simulink model "Project26"  (R2023b)
settings: Solver=ode4  StartTime=0.0  StopTime=4*pi/n  FixedStep=0.1  RelTol=1e-3
values from neighbouring files (symbols this model uses):
  A = [A1; A2; A3; A4; A5; A6; A7; A8; A9; A10; A11; A12; A13; A14]    [Main.m]
  a = (509.4*1000+R_E+529.9*1000+R_E)/2    [Main.m]
  A_ssb = zeros(3,3,6)    [Main.m]
  e = 0.00149    [Main.m]
  epsilon = deg2rad(23.45)    [Main.m]
  F_e = 1358+600+150    (= 2108)    [Main.m]
  FOV = deg2rad(114)    [Main.m]
  G = 6.67*10^-11    (= 6.67e-11)    [Main.m]
  I = [Ix 0 0; 0 Iy 0; 0 0 Iz]    [Main.m]
  i = deg2rad(97.525)    [Main.m]
  I_inv = inv(I)    [Main.m]
  Ix = 0.13    [Main.m]
  Iy = 0.16    [Main.m]
  Iz = 0.18    [Main.m]
  j_B = [0.01, 0.05, 0.01]'    [Main.m]
  Mt = 5.97219e24    (= 5.97219e+24)    [Main.m]
  n = sqrt(G*Mt/a^3)    [Main.m]
  N_B = [n1; n2; n3; n4; n5; n6; n7; n8; n9; n10;n11;n12;n13;n14]    [Main.m]
  n_sun = 2*pi/T_earth    (= 1.99238499086e-07)    [Main.m]
  OM = deg2rad(6.934*180/12)    [Main.m]
  om = deg2rad(287.373)    [Main.m]
  q0 = [0 0 0 1]    [Main.m]
  r_CG = [0.02 0 0]    [Main.m]
  R_sun = astroConstants(2)*1e3    [Main.m]
  rF = [rF1; rF2; rF3; rF4; rF5; rF6; rF7; rF8; rF9; rF10;rF11;rF12;rF13;rF14]    [Main.m]
  theta0 = 0    [Main.m]
  Tsample = 0.1    [Main.m]
  w0 = [w_x0 w_y0 w_z0]    [Main.m]
  w_E = 7.291597763887421e-05    (= 7.29159776389e-05)    [Main.m]
  w_LN = [0 0 n]    [Main.m]
undefined symbols (not defined in the file or in its folder): actuators, control, DiscIntNeverNeededParam, environment, magnitude, sensors, settings
libraries: vrlib x6, matrix_library x5, simulink x2, aerolibutil x1
(part 2 of 2)

== system Project26/Disturbing Torques/Magnetic Torque/Rotation from Inertial to Body Frame ==
  note: $\vec{B_B} = q_{BN}'\otimes [\vec{B_N};0]\otimes q_{BN}$
  note: Quaternion Rotation (Double Tensor Product)
  q_BN : Inport
  B_N : Inport  Port=2
  Demux : Demux
  Mux : Mux  Inputs=3
  Quaternion multiplication 2 : Subsystem
  Quaternion multiplication1 : Subsystem
  To Workspace : ToWorkspace  VariableName=B_B  SampleTime=-1
  Transformation in Quaternion : Subsystem
  Transpose : Gain  Gain=[-1 -1 -1 1]
  B_B : Outport
  wires:
  B_N/1 -> Transformation in Quaternion/1(B_N)
  Mux/1 -> To Workspace/1, B_B/1
  Transpose/1 -> Quaternion multiplication1/1(q_BN)
  q_BN/1 -> Quaternion multiplication 2/2(q_BN), Transpose/1
  Transformation in Quaternion/1(q(B_N)) -> Quaternion multiplication1/2(q(B_N))
  Quaternion multiplication 2/1(q(B_B)) -> Demux/1
  Quaternion multiplication1/1(q1) -> Quaternion multiplication 2/1(q1)
  Demux/1 -> Mux/1
  Demux/2 -> Mux/2
  Demux/3 -> Mux/3

== system Project26/Kinematics/Quaternions/OMEGA Matrix ==
  note: Angular velocity
      | components
  w : Inport
  Demux : Demux  Outputs=3
  Gain1 : Gain  Gain=[0 0 0 1; 0 0 1 0; 0 -1 0 0; -1 0 0 0]
  Gain2 : Gain  Gain=[0 0 -1 0; 0 0 0 1; 1 0 0 0; 0 -1 0 0]
  Gain3 : Gain  Gain=[0 1 0 0; -1 0 0 0; 0 0 0 1; 0 0 -1 0]
  Sum : Sum  Inputs=+++
  OM Matrix : Outport
  wires:
  w/1 -> Demux/1
  Sum/1 -> OM Matrix/1
  Gain3/1 -> Sum/3
  Gain1/1 -> Sum/1
  Demux/2 -> Gain2/1
  Demux/1 -> Gain1/1
  Gain2/1 -> Sum/2
  Demux/3 -> Gain3/1

== system Project26/Orbital Mechanics and Attitude Error / Rotation from Inertial to Body Frame/Quaternion multiplication 1 ==
  q_BN' : Inport
  "q(r_N) " : Inport  Port=2
  Demux : Demux
  Gain : Gain  Gain=[1 0 0 0; 0 1 0 0; 0 0 1 0; 0 0 0 1]
  Gain1 : Gain  Gain=[0 0 0 1; 0 0 1 0 ;0 -1 0 0; -1 0 0 0]
  Gain2 : Gain  Gain=[0 0 -1 0; 0 0 0 1; 1 0 0 0; 0 -1 0 0]
  Gain3 : Gain  Gain=[0 1 0 0; -1 0 0 0; 0 0 0 1; 0 0 -1 0]
  Product : Product  Multiplication=Matrix(*)
  Sum : Sum  Inputs=|++++
  q1 : Outport
  wires:
  "q(r_N) "/1 -> Demux/1
  Demux/4 -> Gain/1
  Demux/1 -> Gain1/1
  Demux/2 -> Gain2/1
  Demux/3 -> Gain3/1
  Gain1/1 -> Sum/1
  Gain2/1 -> Sum/2
  Gain3/1 -> Sum/3
  Gain/1 -> Sum/4
  q_BN'/1 -> Product/2
  Sum/1 -> Product/1
  Product/1 -> q1/1

== system Project26/Orbital Mechanics and Attitude Error / Rotation from Inertial to Body Frame/Quaternion multiplication 2 ==
  q1 : Inport
  q_BN : Inport  Port=2
  Demux : Demux
  Gain : Gain  Gain=[1 0 0 0;0 1 0 0;0 0 1 0; 0 0 0 1]
  Gain1 : Gain  Gain=[0 0 0 1;0 0 1 0;0 -1 0 0;-1 0 0 0]
  Gain2 : Gain  Gain=[0 0 -1 0;0 0 0 1;1 0 0 0;0 -1 0 0]
  Gain3 : Gain  Gain=[0 1 0 0;-1 0 0 0;0 0 0 1;0 0 -1 0]
  Product : Product  Multiplication=Matrix(*)
  Sum : Sum  Inputs=|++++
  q(r_B) : Outport
  wires:
  q_BN/1 -> Demux/1
  Demux/4 -> Gain/1
  Demux/1 -> Gain1/1
  Demux/2 -> Gain2/1
  Demux/3 -> Gain3/1
  Gain1/1 -> Sum/1
  Gain2/1 -> Sum/2
  Gain3/1 -> Sum/3
  Gain/1 -> Sum/4
  q1/1 -> Product/2
  Sum/1 -> Product/1
  Product/1 -> q(r_B)/1

== system Project26/Orbital Mechanics and Attitude Error / Rotation from Inertial to Body Frame/Transformation in Quaternion ==
  note: Adding 0 as fourth element
      | to match the Quaternion's dimensions
  r_N : Inport
  Constant : Constant  Value=0
  Demux : Demux  Outputs=3
  Mux : Mux
  q(r_N) : Outport
  wires:
  r_N/1 -> Demux/1
  Mux/1 -> q(r_N)/1
  Constant/1 -> Mux/4
  Demux/3 -> Mux/3
  Demux/2 -> Mux/2
  Demux/1 -> Mux/1

== system Project26/Orbital Mechanics and Attitude Error /Attitude Error/Computation of q_BL ==
  note: $q_{BL} = q_{LN}'\otimes q_{BN}$
  note: Components of q_LN
  note: Tensor product to compute the error
  q_BN : Inport
  q_LN' : Inport  Port=2
  Demux : Demux
  Gain : Gain  Gain=[0,0,0,-1; 0,0,1,0; 0,-1,0,0; 1,0,0,0]
  Gain1 : Gain  Gain=[0,0,-1,0; 0,0,0,-1; 1,0,0,0; 0,1,0,0]
  Gain2 : Gain  Gain=[0, 1, 0, 0; -1, 0, 0, 0; 0, 0, 0, -1; 0, 0, 1, 0]
  Gain3 : Gain  Gain=[1,0,0,0; 0,1,0,0; 0,0,1,0; 0,0,0,1]
  Product : Product  Multiplication=Matrix(*)
  Sum : Sum  Inputs=|++++
  q_BL : Outport
  wires:
  q_LN'/1 -> Demux/1
  Demux/1 -> Gain/1
  Demux/2 -> Gain1/1
  Demux/3 -> Gain2/1
  Demux/4 -> Gain3/1
  Gain/1 -> Sum/1
  Gain1/1 -> Sum/2
  Gain2/1 -> Sum/3
  Gain3/1 -> Sum/4
  Sum/1 -> Product/1
  q_BN/1 -> Product/2
  Product/1 -> q_BL/1

== system Project26/Orbital Mechanics and Attitude Error /Attitude Error/Rotation of w_LN ==
  note: Quaternion Rotation (Double Tensor Product)
  q_BL : Inport
  w_LN : Inport  Port=2
  Demux : Demux
  Mux : Mux  Inputs=3
  Quaternion multiplication 1 : Subsystem
  Quaternion multiplication 2 : Subsystem
  To Workspace : ToWorkspace  VariableName=w_LN_B  SampleTime=-1
  Transformation in Quaternion : Subsystem
  Transpose : Gain  Gain=[-1 -1 -1 1]
  w_LN' : Outport
  wires:
  w_LN/1 -> Transformation in Quaternion/1(w_LN)
  Mux/1 -> To Workspace/1, w_LN'/1
  Transpose/1 -> Quaternion multiplication 1/1(q_BL')
  q_BL/1 -> Quaternion multiplication 2/2("q_BL "), Transpose/1
  Transformation in Quaternion/1(q_LN) -> Quaternion multiplication 1/2(q_LN)
  Quaternion multiplication 2/1(q(w_LN')) -> Demux/1
  Quaternion multiplication 1/1(q1) -> Quaternion multiplication 2/1(q1)
  Demux/1 -> Mux/1
  Demux/2 -> Mux/2
  Demux/3 -> Mux/3

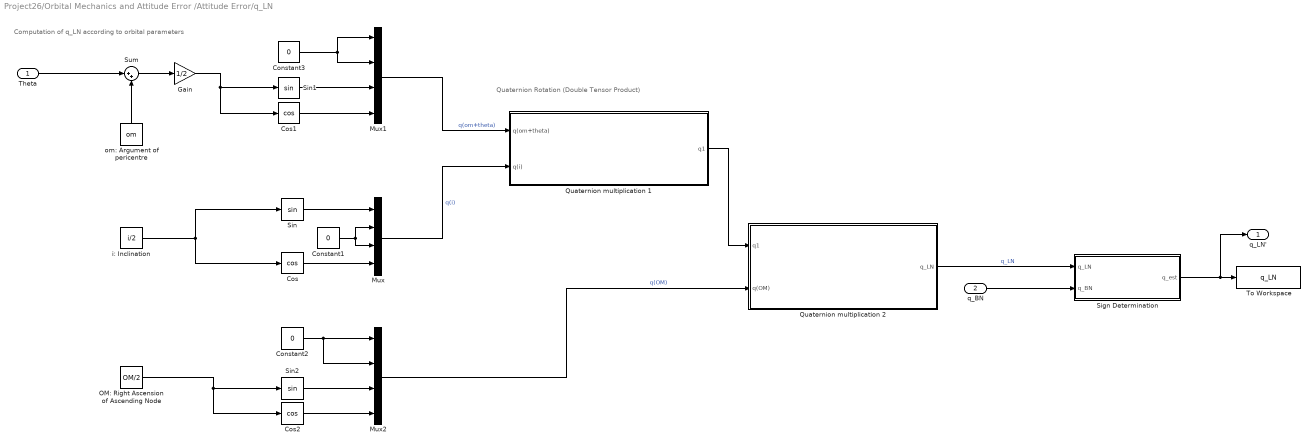
== system Project26/Orbital Mechanics and Attitude Error /Attitude Error/q_LN ==
  note: Quaternion Rotation (Double Tensor Product)
  note: Computation of q_LN according to orbital parameters
  Theta : Inport
  q_BN : Inport  Port=2
  Constant1 : Constant  Value=0
  Constant2 : Constant  Value=0
  Constant3 : Constant  Value=0
  Cos : Trigonometry  Operator=cos
  Cos1 : Trigonometry  Operator=cos
  Cos2 : Trigonometry  Operator=cos
  Gain : Gain  Gain=1/2
  Mux : Mux
  Mux1 : Mux
  Mux2 : Mux
  OM: Right Ascension of Ascending Node : Constant  Value=OM/2
  Quaternion multiplication 1 : Subsystem
  Quaternion multiplication 2 : Subsystem
  Sign Determination : Subsystem
  Sin : Trigonometry
  Sin1 : Trigonometry
  Sin2 : Trigonometry
  Sum : Sum  Inputs=|++
  To Workspace : ToWorkspace  VariableName=q_LN  SampleTime=-1
  i: Inclination : Constant  Value=i/2
  om: Argument of pericentre : Constant  Value=om
  q_LN' : Outport
  wires:
  Cos/1 -> Mux/4
  Sin/1 -> Mux/1
  Constant1/1 -> Mux/2, Mux/3
  Cos1/1 -> Mux1/4
  Constant3/1 -> Mux1/1, Mux1/2
  Sin1/1 -> Mux1/3
  Gain/1 -> Sin1/1, Cos1/1
  i: Inclination/1 -> Cos/1, Sin/1
  Theta/1 -> Sum/1
  Cos2/1 -> Mux2/4
  OM: Right Ascension of Ascending Node/1 -> Cos2/1, Sin2/1
  Sin2/1 -> Mux2/3
  Constant2/1 -> Mux2/2, Mux2/1
  om: Argument of pericentre/1 -> Sum/2
  Sum/1 -> Gain/1
  Mux1/1 -> Quaternion multiplication 1/1(q(om+theta))  "q(om+theta)"
  Mux/1 -> Quaternion multiplication 1/2(q(i))  "q(i)"
  Quaternion multiplication 1/1(q1) -> Quaternion multiplication 2/1(q1)
  Mux2/1 -> Quaternion multiplication 2/2(q(OM))  "q(OM)"
  Quaternion multiplication 2/1(q_LN) -> Sign Determination/1("q_LN ")  "q_LN"
  Sign Determination/1(q_est) -> q_LN'/1, To Workspace/1
  q_BN/1 -> Sign Determination/2(q_BN)

== system Project26/Orbital Mechanics and Attitude Error /Computation of r (vector)/Rotation (R313') from Perifocal to ECI ==
  note: $R_{313}(\Omega,i,\omega) = R_3(\omega) R_1(i)R_3(\Omega)$
  Matrix Multiply : Product  Multiplication=Matrix(*)
  Matrix Multiply1 : Product  Multiplication=Matrix(*)
  R1(i) : Constant  Value=[1 0 0;0 cos(i) sin(i) ;0 -sin(i) cos(i)]
  R3(OM) : Constant  Value=[cos(OM) sin(OM) 0; -sin(OM) cos(OM) 0; 0 0 1]
  R3(om) : Constant  Value=[cos(om) sin(om) 0;-sin(om) cos(om) 0;0 0 1]
  Transpose : Math  Operator=transpose
  Transpose1 : Math  Operator=transpose
  Transpose2 : Math  Operator=transpose
  R313 : Outport
  wires:
  R3(om)/1 -> Transpose/1
  R3(OM)/1 -> Transpose1/1
  R1(i)/1 -> Transpose2/1
  Matrix Multiply1/1 -> R313/1
  Transpose1/1 -> Matrix Multiply/1
  Transpose2/1 -> Matrix Multiply/2
  Matrix Multiply/1 -> Matrix Multiply1/1
  Transpose/1 -> Matrix Multiply1/2

== system Project26/Orbital Mechanics and Attitude Error /Rotation from Inertial to Body Frame/Quaternion multiplication 1 ==
  q_BN' : Inport
  q(S_N) : Inport  Port=2
  Demux : Demux
  Gain : Gain  Gain=[1 0 0 0; 0 1 0 0; 0 0 1 0; 0 0 0 1]
  Gain1 : Gain  Gain=[0 0 0 1; 0 0 1 0; 0 -1 0 0; -1 0 0 0]
  Gain2 : Gain  Gain=[0 0 -1 0; 0 0 0 1; 1 0 0 0; 0 -1 0 0]
  Gain3 : Gain  Gain=[0 1 0 0; -1 0 0 0; 0 0 0 1; 0 0 -1 0]
  Product : Product  Multiplication=Matrix(*)
  Sum : Sum  Inputs=|++++
  q1 : Outport
  wires:
  q(S_N)/1 -> Demux/1
  Demux/4 -> Gain/1
  Demux/1 -> Gain1/1
  Demux/2 -> Gain2/1
  Demux/3 -> Gain3/1
  Gain1/1 -> Sum/1
  Gain2/1 -> Sum/2
  Gain3/1 -> Sum/3
  Gain/1 -> Sum/4
  q_BN'/1 -> Product/2
  Sum/1 -> Product/1
  Product/1 -> q1/1

== system Project26/Orbital Mechanics and Attitude Error /Rotation from Inertial to Body Frame/Quaternion multiplication 2 ==
  q1 : Inport
  q_BN : Inport  Port=2
  Demux : Demux
  Gain : Gain  Gain=[1 0 0 0; 0 1 0 0; 0 0 1 0; 0 0 0 1]
  Gain1 : Gain  Gain=[0 0 0 1; 0 0 1 0; 0 -1 0 0; -1 0 0 0]
  Gain2 : Gain  Gain=[0 0 -1 0; 0 0 0 1; 1 0 0 0; 0 -1 0 0]
  Gain3 : Gain  Gain=[0 1 0 0; -1 0 0 0; 0 0 0 1; 0 0 -1 0]
  Product : Product  Multiplication=Matrix(*)
  Sum : Sum  Inputs=|++++
  q(S_B) : Outport
  wires:
  q_BN/1 -> Demux/1
  Demux/4 -> Gain/1
  Demux/1 -> Gain1/1
  Demux/2 -> Gain2/1
  Demux/3 -> Gain3/1
  Gain1/1 -> Sum/1
  Gain2/1 -> Sum/2
  Gain3/1 -> Sum/3
  Gain/1 -> Sum/4
  q1/1 -> Product/2
  Sum/1 -> Product/1
  Product/1 -> q(S_B)/1

== system Project26/Orbital Mechanics and Attitude Error /Rotation from Inertial to Body Frame/Transformation in Quaternion ==
  note: Adding 0 as fourth element
      | to match the Quaternion's dimensions
  S_N : Inport
  Constant : Constant  Value=0
  Demux : Demux  Outputs=3
  Mux : Mux
  q(S_N) : Outport
  wires:
  S_N/1 -> Demux/1
  Mux/1 -> q(S_N)/1
  Constant/1 -> Mux/4
  Demux/3 -> Mux/3
  Demux/2 -> Mux/2
  Demux/1 -> Mux/1

== system Project26/Sensors/Gyroscopes/Misalignment Error ==
  note: Components
  w_BN : Inport
  Cos (1) : Gain  Gain=cos(sensors.gyro.mys)
  Cos (2) : Gain  Gain=cos(sensors.gyro.mys)
  Cos (3) : Gain  Gain=cos(sensors.gyro.mys)
  Demux : Demux  Outputs=3
  Mux : Mux  Inputs=3
  Sin (1) : Gain  Gain=sin(sensors.gyro.mys/2)
  Sin (2) : Gain  Gain=sin(sensors.gyro.mys/2)
  Sin (3) : Gain  Gain=sin(sensors.gyro.mys/2)
  Sum : Sum  Inputs=|+++
  Sum1 : Sum  Inputs=|+++
  Sum2 : Sum  Inputs=|+++
  w (True Value) : Outport
  wires:
  w_BN/1 -> Demux/1
  Demux/1 -> Sin (1)/1, Cos (1)/1
  Demux/2 -> Sin (2)/1, Cos (2)/1
  Demux/3 -> Cos (3)/1, Sin (3)/1
  Cos (1)/1 -> Sum/1
  Sin (2)/1 -> Sum/2, Sum2/3
  Sin (3)/1 -> Sum/3, Sum1/3
  Cos (2)/1 -> Sum1/1
  Sin (1)/1 -> Sum2/2, Sum1/2
  Cos (3)/1 -> Sum2/1
  Sum1/1 -> Mux/2
  Sum2/1 -> Mux/3
  Sum/1 -> Mux/1
  Mux/1 -> w (True Value)/1

== system Project26/Sensors/Magnetometer/Non-Orthogonality Error ==
  note: Components
  B_B : Inport
  Cos (1) : Gain  Gain=cos(sensors.mag.mys1)
  Cos (2) : Gain  Gain=cos(sensors.mag.mys1)
  Cos (3) : Gain  Gain=cos(sensors.mag.mys1)
  Demux : Demux  Outputs=3
  Mux : Mux  Inputs=3
  Sin (1) : Gain  Gain=sin(sensors.mag.mys2)
  Sin (2) : Gain  Gain=sin(sensors.mag.mys2)
  Sin (3) : Gain  Gain=sin(sensors.mag.mys2)
  Sum : Sum  Inputs=|+++
  Sum1 : Sum  Inputs=|+++
  Sum2 : Sum  Inputs=|+++
  B_B (True) : Outport
  wires:
  B_B/1 -> Demux/1
  Demux/1 -> Cos (1)/1, Sin (1)/1
  Demux/2 -> Sin (2)/1, Cos (2)/1
  Demux/3 -> Cos (3)/1, Sin (3)/1
  Cos (1)/1 -> Sum/1
  Sin (2)/1 -> Sum2/3, Sum/2
  Sin (3)/1 -> Sum1/3, Sum/3
  Cos (2)/1 -> Sum1/1
  Sin (1)/1 -> Sum2/2, Sum1/2
  Cos (3)/1 -> Sum2/1
  Sum1/1 -> Mux/2
  Sum2/1 -> Mux/3
  Sum/1 -> Mux/1
  Mux/1 -> B_B (True)/1

== system Project26/Sensors/Sun Sensor/Angle errors ==
  alpha_x : Inport
  alpha_y : Inport  Port=2
  alpha_z : Inport  Port=3
  Constant1 : Constant  Value=[1 0 0; 0 1 0; 0 0 1]
  Gain5 : Gain  Gain=[0 0 0; 0 0 1; 0 -1 0]
  Gain6 : Gain  Gain=[0 0 -1; 0 0 0; 1 0 0]
  Gain7 : Gain  Gain=[0 1 0; -1 0 0; 0 0 0]
  Sum : Sum  Inputs=|++++
  alpha_err : Outport
  wires:
  Gain7/1 -> Sum/3
  alpha_y/1 -> Gain6/1
  Gain5/1 -> Sum/1
  alpha_x/1 -> Gain5/1
  Constant1/1 -> Sum/4
  Sum/1 -> alpha_err/1
  Gain6/1 -> Sum/2
  alpha_z/1 -> Gain7/1

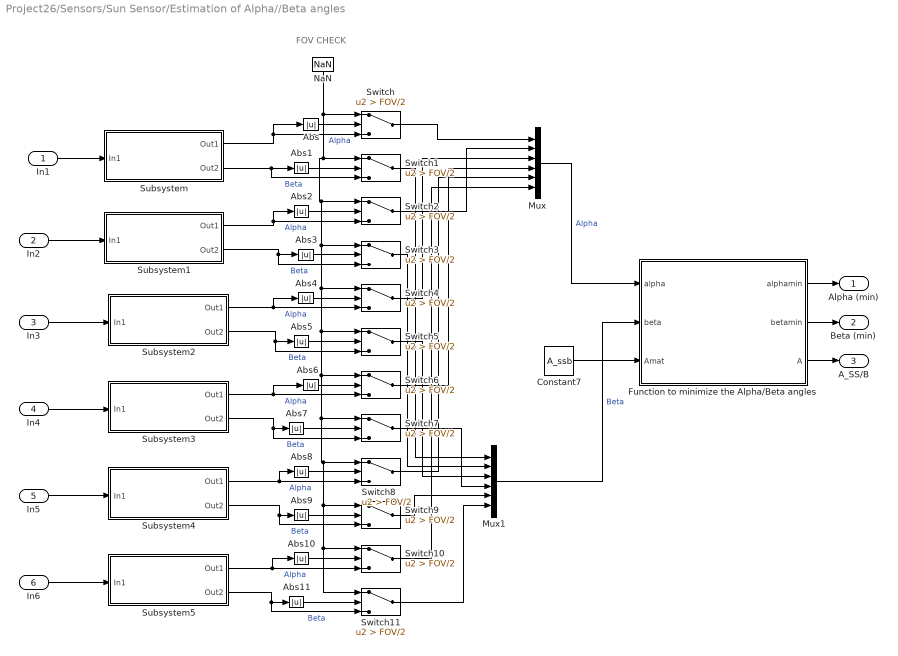
== system Project26/Sensors/Sun Sensor/Estimation of Alpha//Beta angles ==
  note: FOV CHECK
  In1 : Inport
  In2 : Inport  Port=2
  In3 : Inport  Port=3
  In4 : Inport  Port=4
  In5 : Inport  Port=5
  In6 : Inport  Port=6
  Abs{,1..11} (12 alike) : Abs  SaturateOnIntegerOverflow=off
  Constant7 : Constant  Value=A_ssb
  Function to minimize the Alpha/Beta angles : MATLAB Function  TreatAsAtomicUnit=on
  Mux : Mux  Inputs=6
  Mux1 : Mux  Inputs=6
  NaN : Constant  Value=NaN  OutDataTypeStr=Inherit: Inherit via back propagation
  Subsystem : Subsystem
  Subsystem1 : Subsystem
  Subsystem2 : Subsystem
  Subsystem3 : Subsystem
  Subsystem4 : Subsystem
  Subsystem5 : Subsystem
  Switch{,1..11} (12 alike) : Switch  Criteria=u2 > Threshold  Threshold=FOV/2  SaturateOnIntegerOverflow=off  InputSameDT=off
  Alpha (min) : Outport
  Beta (min) : Outport  Port=2
  A_SS/B : Outport  Port=3
  wires:
  Subsystem1/1(Out1) -> Abs2/1, Switch2/3  "Alpha"
  Switch6/1 -> Mux/4
  Subsystem/2(Out2) -> Switch1/3, Abs1/1  "Beta"
  In5/1 -> Subsystem4/1(In1)
  Abs10/1 -> Switch10/2
  Subsystem4/1(Out1) -> Abs8/1, Switch8/3  "Alpha"
  Abs2/1 -> Switch2/2
  Subsystem2/1(Out1) -> Abs4/1, Switch4/3  "Alpha"
  Subsystem3/1(Out1) -> Abs6/1, Switch6/3  "Alpha"
  Switch1/1 -> Mux1/1
  Abs8/1 -> Switch8/2
  Switch5/1 -> Mux1/3
  Mux/1 -> Function to minimize the Alpha/Beta angles/1(alpha)  "Alpha"
  Switch9/1 -> Mux1/5
  Subsystem2/2(Out2) -> Abs5/1, Switch5/3  "Beta"
  Abs3/1 -> Switch3/2
  Subsystem1/2(Out2) -> Abs3/1, Switch3/3  "Beta"
  Subsystem4/2(Out2) -> Switch9/3, Abs9/1  "Beta"
  Switch11/1 -> Mux1/6
  Abs6/1 -> Switch6/2
  Switch3/1 -> Mux1/2
  Abs11/1 -> Switch11/2
  Abs1/1 -> Switch1/2
  In2/1 -> Subsystem1/1(In1)
  NaN/1 -> Switch11/1, Switch10/1, Switch9/1, Switch8/1, Switch7/1, Switch6/1, Switch5/1, Switch4/1, Switch3/1, Switch2/1, Switch1/1, Switch/1
  Subsystem/1(Out1) -> Abs/1, Switch/3  "Alpha"
  Abs4/1 -> Switch4/2
  Subsystem3/2(Out2) -> Switch7/3, Abs7/1  "Beta"
  Subsystem5/1(Out1) -> Abs10/1, Switch10/3  "Alpha"
  Switch8/1 -> Mux/5
  Subsystem5/2(Out2) -> Switch11/3, Abs11/1  "Beta"
  Switch7/1 -> Mux1/4
  In6/1 -> Subsystem5/1(In1)
  Abs9/1 -> Switch9/2
  Switch2/1 -> Mux/2
  Abs7/1 -> Switch7/2
  Abs5/1 -> Switch5/2
  Switch4/1 -> Mux/3
  Switch/1 -> Mux/1
  Abs/1 -> Switch/2
  Switch10/1 -> Mux/6
  In1/1 -> Subsystem/1(In1)
  Mux1/1 -> Function to minimize the Alpha/Beta angles/2(beta)  "Beta"
  In4/1 -> Subsystem3/1(In1)
  In3/1 -> Subsystem2/1(In1)
  Function to minimize the Alpha/Beta angles/1(alphamin) -> Alpha (min)/1
  Constant7/1 -> Function to minimize the Alpha/Beta angles/3(Amat)
  Function to minimize the Alpha/Beta angles/2(betamin) -> Beta (min)/1
  Function to minimize the Alpha/Beta angles/3(A) -> A_SS/B/1

== system Project26/Attitude Determination/Enabled Subsystem/Kinematics/Quaternion ==
  note: Normalized
      | Quaternion
  w : Inport
  q_0 : Inport  Port=2
  q_BN : Inport  Port=3
  Discrete-Time Integrator : DiscreteIntegrator  InitialConditionSource=external  SampleTime=Tsample  ICPrevOutput=DiscIntNeverNeededParam  ICPrevScaledInput=DiscIntNeverNeededParam
  Gain : Gain  Gain=1/2
  Matrix Multiply : Product  Multiplication=Matrix(*)
  Omega Matrix : Subsystem
  To Workspace : ToWorkspace  VariableName=int  SampleTime=-1
  q(t) : Outport
  wires:
  Matrix Multiply/1 -> Discrete-Time Integrator/1
  Gain/1 -> Matrix Multiply/1
  w/1 -> Omega Matrix/1(In1)
  Omega Matrix/1(Out1) -> Gain/1
  q_BN/1 -> Matrix Multiply/2
  Discrete-Time Integrator/1 -> To Workspace/1, q(t)/1
  q_0/1 -> Discrete-Time Integrator/2

== system Project26/Attitude Determination/Enabled Subsystem/Kinematics/Quaternion Normalization ==
  q(t) : Inport
  Divide : Product  Inputs=*/
  Dot Product : DotProduct  OutDataTypeStr=Inherit: Inherit via internal rule
  Sqrt : Sqrt
  q_BN : Outport
  wires:
  Dot Product/1 -> Sqrt/1
  q(t)/1 -> Divide/1, Dot Product/1, Dot Product/2
  Sqrt/1 -> Divide/2
  Divide/1 -> q_BN/1

== system Project26/Attitude Determination/Enabled Subsystem/Sign Determination/Subsystem ==
  q_est : Inport
  Demux : Demux
  Mux : Mux
  Out1 : Outport
  wires:
  q_est/1 -> Demux/1
  Demux/1 -> Mux/1
  Demux/2 -> Mux/2
  Demux/3 -> Mux/3
  Demux/4 -> Mux/4
  Mux/1 -> Out1/1

== system Project26/Attitude Determination/Enabled Subsystem1/Sign determination/Subsystem ==
  q_est : Inport
  Demux : Demux
  Mux : Mux
  Out1 : Outport
  wires:
  q_est/1 -> Demux/1
  Demux/1 -> Mux/1
  Demux/2 -> Mux/2
  Demux/3 -> Mux/3
  Demux/4 -> Mux/4
  Mux/1 -> Out1/1

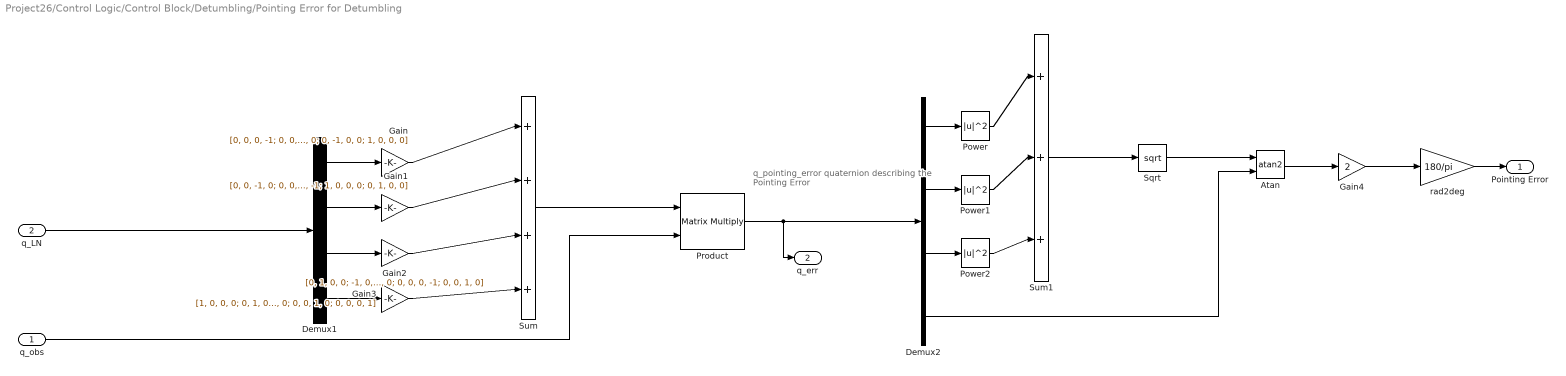
== system Project26/Control Logic/Control Block/Detumbling/Pointing Error for Detumbling ==
  note: q_pointing_error
      | quaternion describing the Pointing Error
  q_obs : Inport
  q_LN : Inport  Port=2
  Atan : Trigonometry  Operator=atan2  OutputSignalType=real
  Demux1 : Demux
  Demux2 : Demux
  Gain : Gain  Gain=[0, 0, 0, -1; 0, 0, 1, 0; 0, -1, 0, 0; 1, 0, 0, 0]
  Gain1 : Gain  Gain=[0, 0, -1, 0; 0, 0, 0, -1; 1, 0, 0, 0; 0, 1, 0, 0]
  Gain2 : Gain  Gain=[0, 1, 0, 0; -1, 0, 0, 0; 0, 0, 0, -1; 0, 0, 1, 0]
  Gain3 : Gain  Gain=[1, 0, 0, 0; 0, 1, 0, 0; 0, 0, 1, 0; 0, 0, 0, 1]
  Gain4 : Gain  Gain=2
  Power : Math  Operator=magnitude^2
  Power1 : Math  Operator=magnitude^2
  Power2 : Math  Operator=magnitude^2
  Product : Product  Multiplication=Matrix(*)
  Sqrt : Sqrt
  Sum : Sum  Inputs=|++++
  Sum1 : Sum  Inputs=|+++
  rad2deg : Gain  Gain=180/pi
  Pointing Error : Outport
  q_err : Outport  Port=2
  wires:
  Power1/1 -> Sum1/2
  Demux2/4 -> Atan/2
  Atan/1 -> Gain4/1
  Power/1 -> Sum1/1
  Demux2/2 -> Power1/1
  Demux2/3 -> Power2/1
  Demux2/1 -> Power/1
  Sum1/1 -> Sqrt/1
  Power2/1 -> Sum1/3
  Sqrt/1 -> Atan/1
  Product/1 -> q_err/1, Demux2/1
  Gain/1 -> Sum/1
  Gain2/1 -> Sum/3
  Gain1/1 -> Sum/2
  Demux1/3 -> Gain2/1
  Demux1/1 -> Gain/1
  Gain3/1 -> Sum/4
  Demux1/2 -> Gain1/1
  Demux1/4 -> Gain3/1
  Sum/1 -> Product/1
  rad2deg/1 -> Pointing Error/1
  q_LN/1 -> Demux1/1
  Gain4/1 -> rad2deg/1
  q_obs/1 -> Product/2

== system Project26/Control Logic/Control Block/Detumbling/Rotation of w_DET ==
  note: Quaternion Rotation (Double Tensor Product)
  w_DET : Inport
  q_err : Inport  Port=2
  Demux : Demux
  Mux : Mux  Inputs=3
  Quaternion multiplication 1 : Subsystem
  Quaternion multiplication 2 : Subsystem
  Transformation in Quaternion : Subsystem
  Transpose : Gain  Gain=[-1 -1 -1 1]
  w_det_body : Outport
  wires:
  w_DET/1 -> Transformation in Quaternion/1(w_LN)
  Mux/1 -> w_det_body/1
  Transpose/1 -> Quaternion multiplication 1/1(q_BL' = q)
  q_err/1 -> Quaternion multiplication 2/2(q_BL = q'), Transpose/1
  Transformation in Quaternion/1(q_LN) -> Quaternion multiplication 1/2(q_LN = q')
  Quaternion multiplication 2/1(q*q' = q2) -> Demux/1
  Quaternion multiplication 1/1(q*q' = q1) -> Quaternion multiplication 2/1(q1 = q)
  Demux/1 -> Mux/1
  Demux/2 -> Mux/2
  Demux/3 -> Mux/3

== system Project26/Control Logic/Control Block/Slew Maneuvre/Pointing Error for Slew Maneuvre ==
  note: q_pointing_error
      | quaternion describing the Pointing Error
  q_LN : Inport
  q_obs : Inport  Port=2
  Atan : Trigonometry  Operator=atan2  OutputSignalType=real
  Demux1 : Demux
  Demux2 : Demux
  Gain : Gain  Gain=[0, 0, 0, -1; 0, 0, 1, 0; 0, -1, 0, 0; 1, 0, 0, 0]
  Gain1 : Gain  Gain=[0, 0, -1, 0; 0, 0, 0, -1; 1, 0, 0, 0; 0, 1, 0, 0]
  Gain2 : Gain  Gain=[0, 1, 0, 0; -1, 0, 0, 0; 0, 0, 0, -1; 0, 0, 1, 0]
  Gain3 : Gain  Gain=[1, 0, 0, 0; 0, 1, 0, 0; 0, 0, 1, 0; 0, 0, 0, 1]
  Gain4 : Gain  Gain=2
  Power : Math  Operator=magnitude^2
  Power1 : Math  Operator=magnitude^2
  Power2 : Math  Operator=magnitude^2
  Product : Product  Multiplication=Matrix(*)
  Sqrt : Sqrt
  Sum : Sum  Inputs=|++++
  Sum1 : Sum  Inputs=|+++
  rad2deg : Gain  Gain=180/pi
  Pointing Error : Outport
  q_e : Outport  Port=2
  wires:
  Power1/1 -> Sum1/2
  Demux2/4 -> Atan/2
  Atan/1 -> rad2deg/1
  Power/1 -> Sum1/1
  Demux2/2 -> Power1/1
  Demux2/3 -> Power2/1
  Demux2/1 -> Power/1
  Sum1/1 -> Sqrt/1
  Power2/1 -> Sum1/3
  Sqrt/1 -> Atan/1
  Product/1 -> Demux2/1, q_e/1
  Gain/1 -> Sum/1
  Gain2/1 -> Sum/3
  Gain1/1 -> Sum/2
  Demux1/3 -> Gain2/1
  Demux1/1 -> Gain/1
  Gain3/1 -> Sum/4
  Demux1/2 -> Gain1/1
  Demux1/4 -> Gain3/1
  Sum/1 -> Product/1
  rad2deg/1 -> Gain4/1
  q_LN/1 -> Demux1/1
  Gain4/1 -> Pointing Error/1
  q_obs/1 -> Product/2

== system Project26/Control Logic/Control Block/Slew Maneuvre/Rotation of w_SM ==
  note: Quaternion Rotation (Double Tensor Product)
  w_SM : Inport
  q_e : Inport  Port=2
  Demux : Demux
  Mux : Mux  Inputs=3
  Quaternion multiplication 1 : Subsystem
  Quaternion multiplication 2 : Subsystem
  Transformation in Quaternion : Subsystem
  Transpose : Gain  Gain=[-1 -1 -1 1]
  w_SM_body : Outport
  wires:
  w_SM/1 -> Transformation in Quaternion/1(w_LN)
  Mux/1 -> w_SM_body/1
  Transpose/1 -> Quaternion multiplication 1/1(q_BL')
  q_e/1 -> Quaternion multiplication 2/2(q_BL), Transpose/1
  Transformation in Quaternion/1(q_LN) -> Quaternion multiplication 1/2(q_LN)
  Quaternion multiplication 2/1(q(w_SM_B)) -> Demux/1
  Quaternion multiplication 1/1(q1) -> Quaternion multiplication 2/1(q1)
  Demux/1 -> Mux/1
  Demux/2 -> Mux/2
  Demux/3 -> Mux/3

== system Project26/Control Logic/Control Block/Trajectory Tracking/Conversion from quaternions to DCM ==
  note: q*q^t
  note: Matrix I
  note: q^tq
  note: q^t
  q_err : Inport
  Demux : Demux
  Gain : Gain  Gain=-2
  Gain1 : Gain  Gain=[1 0 0;0 1 0;0 0 1]
  Gain2 : Gain  Gain=2
  Matrix Multiply : Product  Multiplication=Matrix(*)
  Mux : Mux  Inputs=3
  Product : Product  Multiplication=Matrix(*)
  Product1 : Product
  Square : Math  Operator=square
  Sum : Sum  Inputs=|-+
  Sum1 : Sum  Inputs=|+++
  Transpose : Math  Operator=transpose
  "[q^] matrix" : Subsystem
  A_e : Outport
  wires:
  q_err/1 -> Demux/1
  Demux/1 -> Mux/1, "[q^] matrix"/1(In1)
  Demux/2 -> Mux/2, "[q^] matrix"/2(In2)
  Demux/4 -> Square/1, Gain/1
  Demux/3 -> Mux/3, "[q^] matrix"/3(In3)
  Square/1 -> Sum/2
  Sum/1 -> Gain1/1
  Gain2/1 -> Sum1/1
  Product1/1 -> Sum1/2
  Gain1/1 -> Sum1/3
  Sum1/1 -> A_e/1
  "[q^] matrix"/1(Out1) -> Product1/2
  Gain/1 -> Product1/1
  Transpose/1 -> Product/1, Matrix Multiply/2
  Product/1 -> Sum/1
  Mux/1 -> Matrix Multiply/1, Product/2, Transpose/1
  Matrix Multiply/1 -> Gain2/1

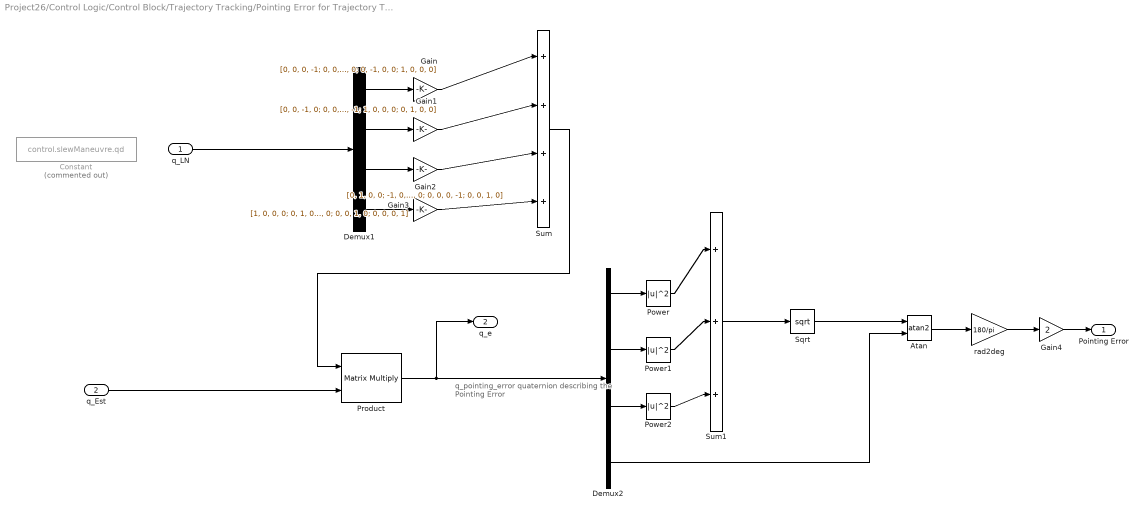
== system Project26/Control Logic/Control Block/Trajectory Tracking/Pointing Error for Trajectory Tracking ==
  note: q_pointing_error
      | quaternion describing the Pointing Error
  q_LN : Inport
  q_Est : Inport  Port=2
  Atan : Trigonometry  Operator=atan2  OutputSignalType=real
  Constant : Constant  Commented=on  Value=control.slewManeuvre.qd
  Demux1 : Demux
  Demux2 : Demux
  Gain : Gain  Gain=[0, 0, 0, -1; 0, 0, 1, 0; 0, -1, 0, 0; 1, 0, 0, 0]
  Gain1 : Gain  Gain=[0, 0, -1, 0; 0, 0, 0, -1; 1, 0, 0, 0; 0, 1, 0, 0]
  Gain2 : Gain  Gain=[0, 1, 0, 0; -1, 0, 0, 0; 0, 0, 0, -1; 0, 0, 1, 0]
  Gain3 : Gain  Gain=[1, 0, 0, 0; 0, 1, 0, 0; 0, 0, 1, 0; 0, 0, 0, 1]
  Gain4 : Gain  Gain=2
  Power : Math  Operator=magnitude^2
  Power1 : Math  Operator=magnitude^2
  Power2 : Math  Operator=magnitude^2
  Product : Product  Multiplication=Matrix(*)
  Sqrt : Sqrt
  Sum : Sum  Inputs=|++++
  Sum1 : Sum  Inputs=|+++
  rad2deg : Gain  Gain=180/pi
  Pointing Error : Outport
  q_e : Outport  Port=2
  wires:
  Power1/1 -> Sum1/2
  Demux2/4 -> Atan/2
  Atan/1 -> rad2deg/1
  Power/1 -> Sum1/1
  Demux2/2 -> Power1/1
  Demux2/3 -> Power2/1
  Demux2/1 -> Power/1
  Sum1/1 -> Sqrt/1
  Power2/1 -> Sum1/3
  Sqrt/1 -> Atan/1
  Product/1 -> Demux2/1, q_e/1
  Gain/1 -> Sum/1
  Gain2/1 -> Sum/3
  Gain1/1 -> Sum/2
  Demux1/3 -> Gain2/1
  Demux1/1 -> Gain/1
  Gain3/1 -> Sum/4
  Demux1/2 -> Gain1/1
  Demux1/4 -> Gain3/1
  Sum/1 -> Product/1
  rad2deg/1 -> Gain4/1
  q_LN/1 -> Demux1/1
  Gain4/1 -> Pointing Error/1
  q_Est/1 -> Product/2

== system Project26/Disturbing Torques/Gravity Gradient Torque/Rotation of vector [1 0 0]/Quaternion multiplication 1 ==
  q_BL : Inport
  q(vect) : Inport  Port=2
  Demux : Demux
  Gain : Gain  Gain=[1 0 0 0; 0 1 0 0; 0 0 1 0; 0 0 0 1]
  Gain1 : Gain  Gain=[0 0 0 1; 0 0 1 0; 0 -1 0 0; -1 0 0 0]
  Gain2 : Gain  Gain=[0 0 -1 0; 0 0 0 1; 1 0 0 0; 0 -1 0 0]
  Gain3 : Gain  Gain=[0 1 0 0; -1 0 0 0; 0 0 0 1; 0 0 -1 0]
  Product : Product  Multiplication=Matrix(*)
  Sum : Sum  Inputs=|++++
  q1 : Outport
  wires:
  q(vect)/1 -> Demux/1
  Demux/4 -> Gain/1
  Demux/1 -> Gain1/1
  Demux/2 -> Gain2/1
  Demux/3 -> Gain3/1
  Gain1/1 -> Sum/1
  Gain2/1 -> Sum/2
  Gain3/1 -> Sum/3
  Gain/1 -> Sum/4
  q_BL/1 -> Product/2
  Sum/1 -> Product/1
  Product/1 -> q1/1

== system Project26/Disturbing Torques/Gravity Gradient Torque/Rotation of vector [1 0 0]/Quaternion multiplication 2 ==
  q1 : Inport
  q_BL : Inport  Port=2
  Demux : Demux
  Gain : Gain  Gain=[1 0 0 0; 0 1 0 0; 0 0 1 0; 0 0 0 1]
  Gain1 : Gain  Gain=[0 0 0 1; 0 0 1 0; 0 -1 0 0; -1 0 0 0]
  Gain2 : Gain  Gain=[0 0 -1 0; 0 0 0 1; 1 0 0 0; 0 -1 0 0]
  Gain3 : Gain  Gain=[0 1 0 0; -1 0 0 0; 0 0 0 1; 0 0 -1 0]
  Product : Product  Multiplication=Matrix(*)
  Sum : Sum  Inputs=|++++
  q(v_rot) : Outport
  wires:
  q_BL/1 -> Demux/1
  Demux/4 -> Gain/1
  Demux/1 -> Gain1/1
  Demux/2 -> Gain2/1
  Demux/3 -> Gain3/1
  Gain1/1 -> Sum/1
  Gain2/1 -> Sum/2
  Gain3/1 -> Sum/3
  Gain/1 -> Sum/4
  q1/1 -> Product/2
  Sum/1 -> Product/1
  Product/1 -> q(v_rot)/1

== system Project26/Disturbing Torques/Gravity Gradient Torque/Rotation of vector [1 0 0]/Transformation in Quaternion ==
  note: Adding 0 as fourth element
      | to match the Quaternion's dimensions
  Vector [1 0 0] : Inport
  Constant : Constant  Value=0
  Demux : Demux  Outputs=3
  Mux : Mux
  q(vect) : Outport
  wires:
  Vector [1 0 0]/1 -> Demux/1
  Mux/1 -> q(vect)/1
  Constant/1 -> Mux/4
  Demux/3 -> Mux/3
  Demux/2 -> Mux/2
  Demux/1 -> Mux/1

== system Project26/Disturbing Torques/Magnetic Torque/Rotation from Inertial to Body Frame/Quaternion multiplication 2 ==
  q1 : Inport
  q_BN : Inport  Port=2
  Demux : Demux
  Gain : Gain  Gain=[1 0 0 0; 0 1 0 0; 0 0 1 0; 0 0 0 1]
  Gain1 : Gain  Gain=[0 0 0 1; 0 0 1 0; 0 -1 0 0; -1 0 0 0]
  Gain2 : Gain  Gain=[0 0 -1 0; 0 0 0 1; 1 0 0 0; 0 -1 0 0]
  Gain3 : Gain  Gain=[0 1 0 0; -1 0 0 0; 0 0 0 1; 0 0 -1 0]
  Product : Product  Multiplication=Matrix(*)
  Sum : Sum  Inputs=|++++
  q(B_B) : Outport
  wires:
  q_BN/1 -> Demux/1
  Demux/4 -> Gain/1
  Demux/1 -> Gain1/1
  Demux/2 -> Gain2/1
  Demux/3 -> Gain3/1
  Gain1/1 -> Sum/1
  Gain2/1 -> Sum/2
  Gain3/1 -> Sum/3
  Gain/1 -> Sum/4
  q1/1 -> Product/2
  Sum/1 -> Product/1
  Product/1 -> q(B_B)/1

== system Project26/Disturbing Torques/Magnetic Torque/Rotation from Inertial to Body Frame/Quaternion multiplication1 ==
  q_BN : Inport
  q(B_N) : Inport  Port=2
  Demux : Demux
  Gain : Gain  Gain=[1 0 0 0; 0 1 0 0; 0 0 1 0; 0 0 0 1]
  Gain1 : Gain  Gain=[0 0 0 1; 0 0 1 0; 0 -1 0 0; -1 0 0 0]
  Gain2 : Gain  Gain=[0 0 -1 0; 0 0 0 1; 1 0 0 0; 0 -1 0 0]
  Gain3 : Gain  Gain=[0 1 0 0; -1 0 0 0; 0 0 0 1; 0 0 -1 0]
  Product : Product  Multiplication=Matrix(*)
  Sum : Sum  Inputs=|++++
  q1 : Outport
  wires:
  q(B_N)/1 -> Demux/1
  Demux/4 -> Gain/1
  Demux/1 -> Gain1/1
  Demux/2 -> Gain2/1
  Demux/3 -> Gain3/1
  Gain1/1 -> Sum/1
  Gain2/1 -> Sum/2
  Gain3/1 -> Sum/3
  Gain/1 -> Sum/4
  q_BN/1 -> Product/2
  Sum/1 -> Product/1
  Product/1 -> q1/1

== system Project26/Disturbing Torques/Magnetic Torque/Rotation from Inertial to Body Frame/Transformation in Quaternion ==
  note: Adding 0 as fourth element
      | to match the Quaternion's dimensions
  B_N : Inport
  Constant : Constant  Value=0
  Demux : Demux  Outputs=3
  Mux : Mux
  q(B_N) : Outport
  wires:
  B_N/1 -> Demux/1
  Mux/1 -> q(B_N)/1
  Constant/1 -> Mux/4
  Demux/3 -> Mux/3
  Demux/2 -> Mux/2
  Demux/1 -> Mux/1

== system Project26/Orbital Mechanics and Attitude Error /Attitude Error/Rotation of w_LN/Quaternion multiplication 1 ==
  q_BL' : Inport
  q_LN : Inport  Port=2
  Demux : Demux
  Gain : Gain  Gain=[1 0 0 0; 0 1 0 0; 0 0 1 0; 0 0 0 1]
  Gain1 : Gain  Gain=[0 0 0 1; 0 0 1 0; 0 -1 0 0; -1 0 0 0]
  Gain2 : Gain  Gain=[0 0 -1 0; 0 0 0 1; 1 0 0 0; 0 -1 0 0]
  Gain3 : Gain  Gain=[0 1 0 0; -1 0 0 0; 0 0 0 1; 0 0 -1 0]
  Product : Product  Multiplication=Matrix(*)
  Sum : Sum  Inputs=|++++
  q1 : Outport
  wires:
  q_LN/1 -> Demux/1
  Demux/4 -> Gain/1
  Demux/1 -> Gain1/1
  Demux/2 -> Gain2/1
  Demux/3 -> Gain3/1
  Gain1/1 -> Sum/1
  Gain2/1 -> Sum/2
  Gain3/1 -> Sum/3
  Gain/1 -> Sum/4
  q_BL'/1 -> Product/2
  Sum/1 -> Product/1
  Product/1 -> q1/1

== system Project26/Orbital Mechanics and Attitude Error /Attitude Error/Rotation of w_LN/Quaternion multiplication 2 ==
  q1 : Inport
  "q_BL " : Inport  Port=2
  Demux : Demux
  Gain : Gain  Gain=[1 0 0 0; 0 1 0 0; 0 0 1 0; 0 0 0 1]
  Gain1 : Gain  Gain=[0 0 0 1;0 0 1 0;0 -1 0 0;-1 0 0 0]
  Gain2 : Gain  Gain=[0 0 -1 0;0 0 0 1;1 0 0 0;0 -1 0 0]
  Gain3 : Gain  Gain=[0 1 0 0; -1 0 0 0; 0 0 0 1; 0 0 -1 0]
  Product : Product  Multiplication=Matrix(*)
  Sum : Sum  Inputs=|++++
  q(w_LN') : Outport
  wires:
  "q_BL "/1 -> Demux/1
  Demux/4 -> Gain/1
  Demux/1 -> Gain1/1
  Demux/2 -> Gain2/1
  Demux/3 -> Gain3/1
  Gain1/1 -> Sum/1
  Gain2/1 -> Sum/2
  Gain3/1 -> Sum/3
  Gain/1 -> Sum/4
  q1/1 -> Product/2
  Sum/1 -> Product/1
  Product/1 -> q(w_LN')/1

== system Project26/Orbital Mechanics and Attitude Error /Attitude Error/Rotation of w_LN/Transformation in Quaternion ==
  note: Adding 0 as fourth element
      | to match the Quaternion's dimension
  w_LN : Inport
  Constant : Constant  Value=0
  Demux : Demux  Outputs=3
  Mux : Mux
  q_LN : Outport
  wires:
  w_LN/1 -> Demux/1
  Mux/1 -> q_LN/1
  Constant/1 -> Mux/4
  Demux/3 -> Mux/3
  Demux/2 -> Mux/2
  Demux/1 -> Mux/1

== system Project26/Orbital Mechanics and Attitude Error /Attitude Error/q_LN/Quaternion multiplication 1 ==
  q(om+theta) : Inport
  q(i) : Inport  Port=2
  Demux : Demux
  Gain : Gain  Gain=[1 0 0 0; 0 1 0 0; 0 0 1 0; 0 0 0 1]
  Gain1 : Gain  Gain=[0 0 0 1; 0 0 1 0; 0 -1 0 0; -1 0 0 0]
  Gain2 : Gain  Gain=[0 0 -1 0; 0 0 0 1; 1 0 0 0; 0 -1 0 0]
  Gain3 : Gain  Gain=[0 1 0 0; -1 0 0 0; 0 0 0 1; 0 0 -1 0]
  Product : Product  Multiplication=Matrix(*)
  Sum : Sum  Inputs=|++++
  q1 : Outport
  wires:
  q(om+theta)/1 -> Demux/1
  Demux/4 -> Gain/1
  Demux/1 -> Gain1/1
  Demux/2 -> Gain2/1
  Demux/3 -> Gain3/1
  Gain1/1 -> Sum/1
  Gain2/1 -> Sum/2
  Gain3/1 -> Sum/3
  Gain/1 -> Sum/4
  q(i)/1 -> Product/2
  Sum/1 -> Product/1
  Product/1 -> q1/1

== system Project26/Orbital Mechanics and Attitude Error /Attitude Error/q_LN/Quaternion multiplication 2 ==
  q1 : Inport
  q(OM) : Inport  Port=2
  Demux : Demux
  Gain : Gain  Gain=[1 0 0 0; 0 1 0 0; 0 0 1 0; 0 0 0 1]
  Gain1 : Gain  Gain=[0 0 0 1; 0 0 1 0; 0 -1 0 0; -1 0 0 0]
  Gain2 : Gain  Gain=[0 0 -1 0; 0 0 0 1; 1 0 0 0; 0 -1 0 0]
  Gain3 : Gain  Gain=[0 1 0 0; -1 0 0 0; 0 0 0 1; 0 0 -1 0]
  Product : Product  Multiplication=Matrix(*)
  Sum : Sum  Inputs=|++++
  q_LN : Outport
  wires:
  q1/1 -> Demux/1
  Demux/4 -> Gain/1
  Demux/1 -> Gain1/1
  Demux/2 -> Gain2/1
  Demux/3 -> Gain3/1
  Gain1/1 -> Sum/1
  Gain2/1 -> Sum/2
  Gain3/1 -> Sum/3
  Gain/1 -> Sum/4
  q(OM)/1 -> Product/2
  Sum/1 -> Product/1
  Product/1 -> q_LN/1

== system Project26/Orbital Mechanics and Attitude Error /Attitude Error/q_LN/Sign Determination ==
  "q_LN " : Inport
  q_BN : Inport  Port=2
  Function to determinate the correct sign of the estimated quaternion : MATLAB Function  TreatAsAtomicUnit=on
  Subsystem : Subsystem
  q_est : Outport
  wires:
  Subsystem/1(Out1) -> q_est/1
  "q_LN "/1 -> Function to determinate the correct sign of the estimated quaternion/2("q_est ")
  q_BN/1 -> Function to determinate the correct sign of the estimated quaternion/1(q_BN)
  Function to determinate the correct sign of the estimated quaternion/1(q_est) -> Subsystem/1(q_est)

== system Project26/Sensors/Sun Sensor/Estimation of Alpha//Beta angles/Subsystem ==
  In1 : Inport
  Atan1 : Trigonometry  Operator=atan2
  Atan2 : Trigonometry  Operator=atan2
  Demux : Demux  Outputs=3
  Out1 : Outport
  Out2 : Outport  Port=2
  wires:
  Demux/3 -> Atan2/2, Atan1/2  "Sz"
  Atan1/1 -> Out2/1
  Demux/1 -> Atan2/1  "Sx"
  In1/1 -> Demux/1
  Demux/2 -> Atan1/1  "Sy"
  Atan2/1 -> Out1/1

== system Project26/Sensors/Sun Sensor/Estimation of Alpha//Beta angles/Subsystem1 ==
  In1 : Inport
  Atan1 : Trigonometry  Operator=atan2
  Atan2 : Trigonometry  Operator=atan2
  Demux : Demux  Outputs=3
  Out1 : Outport
  Out2 : Outport  Port=2
  wires:
  Demux/3 -> Atan2/2, Atan1/2  "Sz"
  Atan1/1 -> Out2/1
  Demux/1 -> Atan2/1  "Sx"
  In1/1 -> Demux/1
  Demux/2 -> Atan1/1  "Sy"
  Atan2/1 -> Out1/1

== system Project26/Sensors/Sun Sensor/Estimation of Alpha//Beta angles/Subsystem2 ==
  In1 : Inport
  Atan1 : Trigonometry  Operator=atan2
  Atan2 : Trigonometry  Operator=atan2
  Demux : Demux  Outputs=3
  Out1 : Outport
  Out2 : Outport  Port=2
  wires:
  Demux/3 -> Atan2/2, Atan1/2  "Sz"
  Atan1/1 -> Out2/1
  Demux/1 -> Atan2/1  "Sx"
  In1/1 -> Demux/1
  Demux/2 -> Atan1/1  "Sy"
  Atan2/1 -> Out1/1

== system Project26/Sensors/Sun Sensor/Estimation of Alpha//Beta angles/Subsystem3 ==
  In1 : Inport
  Atan1 : Trigonometry  Operator=atan2
  Atan2 : Trigonometry  Operator=atan2
  Demux : Demux  Outputs=3
  Out1 : Outport
  Out2 : Outport  Port=2
  wires:
  Demux/3 -> Atan2/2, Atan1/2  "Sz"
  Atan1/1 -> Out2/1
  Demux/1 -> Atan2/1  "Sx"
  In1/1 -> Demux/1
  Demux/2 -> Atan1/1  "Sy"
  Atan2/1 -> Out1/1

== system Project26/Sensors/Sun Sensor/Estimation of Alpha//Beta angles/Subsystem4 ==
  In1 : Inport
  Atan1 : Trigonometry  Operator=atan2
  Atan2 : Trigonometry  Operator=atan2
  Demux : Demux  Outputs=3
  Out1 : Outport
  Out2 : Outport  Port=2
  wires:
  Demux/3 -> Atan2/2, Atan1/2  "Sz"
  Atan1/1 -> Out2/1
  Demux/1 -> Atan2/1  "Sx"
  In1/1 -> Demux/1
  Demux/2 -> Atan1/1  "Sy"
  Atan2/1 -> Out1/1

== system Project26/Sensors/Sun Sensor/Estimation of Alpha//Beta angles/Subsystem5 ==
  In1 : Inport
  Atan1 : Trigonometry  Operator=atan2
  Atan2 : Trigonometry  Operator=atan2
  Demux : Demux  Outputs=3
  Out1 : Outport
  Out2 : Outport  Port=2
  wires:
  Demux/3 -> Atan2/2, Atan1/2  "Sz"
  Atan1/1 -> Out2/1
  Demux/1 -> Atan2/1  "Sx"
  In1/1 -> Demux/1
  Demux/2 -> Atan1/1  "Sy"
  Atan2/1 -> Out1/1

== system Project26/Attitude Determination/Enabled Subsystem/Kinematics/Quaternion/Omega Matrix ==
  note: Angular Velocity
      | Components
  In1 : Inport
  Demux : Demux  Outputs=3
  Gain1 : Gain  Gain=[0 0 0 1; 0 0 1 0; 0 -1 0 0; -1 0 0 0]
  Gain2 : Gain  Gain=[0 0 -1 0; 0 0 0 1; 1 0 0 0; 0 -1 0 0]
  Gain3 : Gain  Gain=[0 1 0 0; -1 0 0 0; 0 0 0 1; 0 0 -1 0]
  Sum : Sum  Inputs=+++
  Out1 : Outport
  wires:
  In1/1 -> Demux/1
  Sum/1 -> Out1/1
  Gain3/1 -> Sum/3
  Gain1/1 -> Sum/1
  Demux/2 -> Gain2/1
  Demux/1 -> Gain1/1
  Gain2/1 -> Sum/2
  Demux/3 -> Gain3/1

== system Project26/Control Logic/Control Block/Detumbling/Rotation of w_DET/Quaternion multiplication 1 ==
  q_BL' = q : Inport
  q_LN = q' : Inport  Port=2
  Demux : Demux
  Gain : Gain  Gain=[1 0 0 0; 0 1 0 0; 0 0 1 0; 0 0 0 1]
  Gain1 : Gain  Gain=[0 0 0 1; 0 0 1 0; 0 -1 0 0; -1 0 0 0]
  Gain2 : Gain  Gain=[0 0 -1 0; 0 0 0 1; 1 0 0 0; 0 -1 0 0]
  Gain3 : Gain  Gain=[0 1 0 0; -1 0 0 0; 0 0 0 1; 0 0 -1 0]
  Product : Product  Multiplication=Matrix(*)
  Sum : Sum  Inputs=|++++
  q*q' = q1 : Outport
  wires:
  q_LN = q'/1 -> Demux/1
  Demux/4 -> Gain/1
  Demux/1 -> Gain1/1
  Demux/2 -> Gain2/1
  Demux/3 -> Gain3/1
  Gain1/1 -> Sum/1
  Gain2/1 -> Sum/2
  Gain3/1 -> Sum/3
  Gain/1 -> Sum/4
  q_BL' = q/1 -> Product/2
  Sum/1 -> Product/1
  Product/1 -> q*q' = q1/1

== system Project26/Control Logic/Control Block/Detumbling/Rotation of w_DET/Quaternion multiplication 2 ==
  q1 = q : Inport
  q_BL = q' : Inport  Port=2
  Demux : Demux
  Gain : Gain  Gain=[1 0 0 0; 0 1 0 0; 0 0 1 0; 0 0 0 1]
  Gain1 : Gain  Gain=[0 0 0 1;0 0 1 0;0 -1 0 0;-1 0 0 0]
  Gain2 : Gain  Gain=[0 0 -1 0;0 0 0 1;1 0 0 0;0 -1 0 0]
  Gain3 : Gain  Gain=[0 1 0 0; -1 0 0 0; 0 0 0 1; 0 0 -1 0]
  Product : Product  Multiplication=Matrix(*)
  Sum : Sum  Inputs=|++++
  q*q' = q2 : Outport
  wires:
  q_BL = q'/1 -> Demux/1
  Demux/4 -> Gain/1
  Demux/1 -> Gain1/1
  Demux/2 -> Gain2/1
  Demux/3 -> Gain3/1
  Gain1/1 -> Sum/1
  Gain2/1 -> Sum/2
  Gain3/1 -> Sum/3
  Gain/1 -> Sum/4
  q1 = q/1 -> Product/2
  Sum/1 -> Product/1
  Product/1 -> q*q' = q2/1

== system Project26/Control Logic/Control Block/Detumbling/Rotation of w_DET/Transformation in Quaternion ==
  note: Adding 0 as fourth element
      | to match the Quaternion's dimension
  w_LN : Inport
  Constant : Constant  Value=0
  Demux : Demux  Outputs=3
  Mux : Mux
  q_LN : Outport
  wires:
  w_LN/1 -> Demux/1
  Mux/1 -> q_LN/1
  Constant/1 -> Mux/4
  Demux/3 -> Mux/3
  Demux/2 -> Mux/2
  Demux/1 -> Mux/1

== system Project26/Control Logic/Control Block/Slew Maneuvre/Rotation of w_SM/Quaternion multiplication 1 ==
  q_BL' : Inport
  q_LN : Inport  Port=2
  Demux : Demux
  Gain : Gain  Gain=[1 0 0 0; 0 1 0 0; 0 0 1 0; 0 0 0 1]
  Gain1 : Gain  Gain=[0 0 0 1; 0 0 1 0; 0 -1 0 0; -1 0 0 0]
  Gain2 : Gain  Gain=[0 0 -1 0; 0 0 0 1; 1 0 0 0; 0 -1 0 0]
  Gain3 : Gain  Gain=[0 1 0 0; -1 0 0 0; 0 0 0 1; 0 0 -1 0]
  Product : Product  Multiplication=Matrix(*)
  Sum : Sum  Inputs=|++++
  q1 : Outport
  wires:
  q_LN/1 -> Demux/1
  Demux/4 -> Gain/1
  Demux/1 -> Gain1/1
  Demux/2 -> Gain2/1
  Demux/3 -> Gain3/1
  Gain1/1 -> Sum/1
  Gain2/1 -> Sum/2
  Gain3/1 -> Sum/3
  Gain/1 -> Sum/4
  q_BL'/1 -> Product/2
  Sum/1 -> Product/1
  Product/1 -> q1/1

== system Project26/Control Logic/Control Block/Slew Maneuvre/Rotation of w_SM/Quaternion multiplication 2 ==
  q1 : Inport
  q_BL : Inport  Port=2
  Demux : Demux
  Gain : Gain  Gain=[1 0 0 0; 0 1 0 0; 0 0 1 0; 0 0 0 1]
  Gain1 : Gain  Gain=[0 0 0 1;0 0 1 0;0 -1 0 0;-1 0 0 0]
  Gain2 : Gain  Gain=[0 0 -1 0;0 0 0 1;1 0 0 0;0 -1 0 0]
  Gain3 : Gain  Gain=[0 1 0 0; -1 0 0 0; 0 0 0 1; 0 0 -1 0]
  Product : Product  Multiplication=Matrix(*)
  Sum : Sum  Inputs=|++++
  q(w_SM_B) : Outport
  wires:
  q_BL/1 -> Demux/1
  Demux/4 -> Gain/1
  Demux/1 -> Gain1/1
  Demux/2 -> Gain2/1
  Demux/3 -> Gain3/1
  Gain1/1 -> Sum/1
  Gain2/1 -> Sum/2
  Gain3/1 -> Sum/3
  Gain/1 -> Sum/4
  q1/1 -> Product/2
  Sum/1 -> Product/1
  Product/1 -> q(w_SM_B)/1

== system Project26/Control Logic/Control Block/Slew Maneuvre/Rotation of w_SM/Transformation in Quaternion ==
  note: Adding 0 as fourth element
      | to match the Quaternion's dimension
  w_LN : Inport
  Constant : Constant  Value=0
  Demux : Demux  Outputs=3
  Mux : Mux
  q_LN : Outport
  wires:
  w_LN/1 -> Demux/1
  Mux/1 -> q_LN/1
  Constant/1 -> Mux/4
  Demux/3 -> Mux/3
  Demux/2 -> Mux/2
  Demux/1 -> Mux/1

== system Project26/Control Logic/Control Block/Trajectory Tracking/Conversion from quaternions to DCM/[q^] matrix ==
  In1 : Inport
  In2 : Inport  Port=2
  In3 : Inport  Port=3
  Gain : Gain  Gain=[0 0 0;0 0 -1;0 1 0]
  Gain1 : Gain  Gain=[0 0 1;0 0 0;-1 0 0]
  Gain2 : Gain  Gain=[0 -1 0;1 0 0;0 0 0]
  Sum : Sum  Inputs=|+++
  Out1 : Outport
  wires:
  In1/1 -> Gain/1
  In2/1 -> Gain1/1
  In3/1 -> Gain2/1
  Gain/1 -> Sum/1
  Gain1/1 -> Sum/2
  Gain2/1 -> Sum/3
  Sum/1 -> Out1/1

== system Project26/Orbital Mechanics and Attitude Error /Attitude Error/q_LN/Sign Determination/Subsystem ==
  q_est : Inport
  Demux : Demux
  Mux : Mux
  Out1 : Outport
  wires:
  q_est/1 -> Demux/1
  Demux/1 -> Mux/1
  Demux/2 -> Mux/2
  Demux/3 -> Mux/3
  Demux/4 -> Mux/4
  Mux/1 -> Out1/1

== matlab function Project26/Disturbing Torques/MATLAB Function2 ==
  data: r_N input; S_N input; S_B input; M_SRP output; F_e input; isEclipse output; A input; N_B input; rf input; r_CG input
function [M_SRP, isEclipse] = fcn(r_N,S_N,S_B, F_e,A,N_B,rf,r_CG)

c = 3e8;
M_SRP = [0; 0; 0];

rho_s = [0.5 0.1]';
rho_d = [0.1 0.1]';

% Determine if the satellite is in Eclipse
R_e = 6378.1*1000;
r_Nnorm=norm(r_N);


if dot(r_N,S_N./norm(S_N))<-sqrt(r_Nnorm^2-R_e^2)
    isEclipse = 1;
    F_e=600+150;
else
    isEclipse=0;
end
P = F_e/c;
    for i = 1:length(N_B)
    N_Bi = N_B(i,:)';
    DOT = dot(S_B,N_Bi);
    if DOT>0
        j = 1;
        if i>6
            j = 2;
        end
        F = -P*A(i)*DOT*((1-rho_s(j))*S_B + (2*rho_s(j)*DOT+2/3*rho_d(j))*N_Bi);
        r = rf(i,:)'- r_CG;
        M_SRP = M_SRP + cross(r,F); 
    end
    end
end

== matlab function Project26/Disturbing Torques/Magnetic Torque/Magnetic Field Model ==
  data: alpha_G input; long input; radius input; B output; lat input; environment parameter; settings parameter
function B = magneticField(alpha_G,long,radius,lat,environment,settings)
% Return the magnetic field component in inertial reference frame

theta = (pi/2-lat); % Colatitude [rad]
alpha = long + alpha_G; 

g = environment.WMM.g;
h = environment.WMM.h;
K = environment.WMM.K;
R = environment.R;
N = settings.N;

%% P-dP
% Validated through the P and dP tables in "Jeremy Davis, Mathematical Modeling of Earth's Magnetic
% Field, 2004"
%%%%%%%%%%%%%%%%%%%%%%%%%%%%%%%%%%%%%%%%%%%%%%%%%%%%%%%%%%%%%%%%%%%%%%%%%%%%%%%%%%%%%%%%%%%%%%%%
% P_{(n),(m+1)}: 
% given P(a,b) -> n=a, m=b-1
% n: from 1 to N
% m: from 0 to N
% N : order of accuracy
%%%%%%%%%%%%%%%%%%%%%%%%%%%%%%%%%%%%%%%%%%%%%%%%%%%%%%%%%%%%%%%%%%%%%%%%%%%%%%%%%%%%%%%%%%%%%%%%

P = zeros(N,N+1);
dP = zeros(N,N+1);

P_00 = 1;
dP_00 = 0;

P_01 = 0; 
dP_01 = 0;

P(1,1) = cos(theta); % n=1, m=0
dP(1,1) = -sin(theta)*P_00; 

P(1,2) = sin(theta);  % n=1, m=1
dP(1,2) = cos(theta)*P_00;

for i = 2:N % Loop in n starting from n = 2 to n = N
    for j = 0:i % Loop in m starting from m = 0 to m = n
        if j == i
        P(i,j+1) = sin(theta)*P(i-1,j);
        dP(i,j+1) = sin(theta)*dP(i-1,j) + cos(theta)*P(i-1,j);
        elseif i < 3
            if j == 0 % n=2, m=0
            P(i,j+1) = cos(theta)*P(i-1,j+1) - K(i,j+1)*P_00;
            dP(i,j+1) = -sin(theta)*P(i-1,j+1) + cos(theta)*dP(i-1,j+1) ...
                - K(i,j+1)*dP_00;
            elseif j == 1 % n=2, m=1
                P(i,j+1) = cos(theta)*P(i-1,j+1) - K(i,j+1)*P_01;
                dP(i,j+1) = -sin(theta)*P(i-1,j+1) + cos(theta)*dP(i-1,j+1)...
                    - K(i,j+1)*dP_01;
            end
        else
            P(i,j+1) = cos(theta)*P(i-1,j+1) - K(i,j+1)*P(i-2,j+1);
            dP(i,j+1) = -sin(theta)*P(i-1,j+1) + cos(theta)*dP(i-1,j+1) ...
                - K(i,j+1)*dP(i-2,j+1);
        end
    end
end

%% Magnetic Field

B_r = 0;
B_th = 0;
B_phi = 0;

% Index i scans n from 1 to N
% Index j scans m from 0 to n

for m = 0:N
    for n = 1:N
        if m<=n
            B_r = B_r + (R/radius)^(n+2)*(n+1)*...
                ((g(n,m+1)*cos(m*long) + h(n,m+1)*sin(m*long))*P(n, m+1));
            B_th = B_th + (R/radius)^(n+2)*...
                ((g(n,m+1)*cos(m*long) + h(n,m+1)*sin(m*long))*dP(n, m+1));
            B_phi = B_phi + (R/radius)^(n+2)*...
                (m*(-g(n,m+1)*sin(m*long) + h(n,m+1)*cos(m*long))* P(n, m+1));

        end

    end
end

B_th = -B_th;
B_phi = -B_phi/sin(theta);

B_x = ( B_r*cos(lat) + B_th*sin(lat) ) * cos(alpha) - B_phi*sin(alpha);
B_y = ( B_r*cos(lat) + B_th*sin(lat) ) * sin(alpha) + B_phi*cos(alpha);
B_z = B_r*sin(lat) - B_th*cos(lat);

B = [B_x B_y B_z]';

== matlab function Project26/Attitude Determination/Enabled Subsystem1/Attitude determination ==
  data: a_mag input; a_sun input; S_N input; q_est output; S_B_Estim input; B_N input; B_B_Estim input
function q_est = q_method(a_mag, a_sun, S_N, S_B_Estim ,B_N, B_B_Estim)

% True measures vector
V_n = [B_N/norm(B_N) S_N];
% Estimated measures vector
Sm_b = [B_B_Estim/norm(B_B_Estim) S_B_Estim];
% Weights vector
a = [1/a_mag 1/a_sun];
a = a./sum(a);
%% Building of matrix K
% Matrix B
B = zeros(3,3);
for i = 1:2
    B = B+a(i)*Sm_b(:,i)*V_n(:,i)';
end

S = B+B';
z = [B(2,3)-B(3,2) B(3,1)-B(1,3) B(1,2)-B(2,1)]';
sigma = trace(B);

K = [S-sigma*eye(3) z;z' sigma];

[Q,L] = eig(K);
[~,index] = max(real(diag(L)));
q_est = real(Q(:,index));

== matlab function Project26/Actuators/MATLAB Function ==
  data: M_RWs input; Msat input; MC_saturation output; w_RWs input; wsat input; h_RWs input; hsat input
function MC_saturation = fcn(M_RWs, Msat, w_RWs, wsat,  h_RWs, hsat)

% Saturation check:

if    abs(h_RWs(1)) > hsat || abs(h_RWs(2)) > hsat || abs(h_RWs(3)) > hsat || ...
      abs(w_RWs(1)) > wsat || abs(w_RWs(2)) > wsat || abs(w_RWs(3)) > wsat || ...
      abs(M_RWs(1)) > Msat || abs(M_RWs(2)) > Msat || abs(M_RWs(3)) > Msat
     
    disp('Reaction Wheel reached saturation'); % Saturation -> attenuation of the required control
end

MC_saturation = zeros(3,1); % No saturation -> no attenuation of the signal

== matlab function Project26/Attitude Determination/Enabled Subsystem/Sign Determination/Function to determinate the correct sign of the estimated quaternion ==
  data: q_BN input; q_est output; q_est input
function q_est = fcn(q_BN,q_est)

[~,index] = max(abs(q_BN));

if q_est(index)*q_BN(index)>0
    q_est = q_est;
else
    q_est = -q_est;
end

== matlab function Project26/Sensors/Sun Sensor/Estimation of Alpha//Beta angles/Function to minimize the Alpha//Beta angles ==
  data: alpha input; alphamin output; betamin output; A output; beta input; Amat input
function [alphamin,betamin,A] = minimum(alpha, beta, Amat)

[~,i] = min(abs(alpha)+abs(beta));
alphamin = alpha(i);
betamin = beta(i);

if i==1
    A=Amat(:,:,1);
elseif i==2
    A=Amat(:,:,2);
elseif i==3
    A=Amat(:,:,3);
elseif i==4
    A=Amat(:,:,4);
elseif i==5
    A=Amat(:,:,5);
else
    A=Amat(:,:,6);
end

end

== matlab function Project26/Attitude Determination/Enabled Subsystem1/Sign determination/Function to determinate the correct sign of the estimated quaternion ==
  data: q_BN input; q_est output; q_est input
function q_est = fcn(q_BN,q_est)

[~,index] = max(abs(q_BN));
if q_est(index)*q_BN(index)>0
    q_est = q_est;
else
    q_est = -q_est;
end

== matlab function Project26/Orbital Mechanics and Attitude Error /Attitude Error/q_LN/Sign Determination/Function to determinate the correct sign of the estimated quaternion ==
  data: q_BN input; q_est output; q_est input
function q_est = fcn(q_BN,q_est)

[~,index] = max(abs(q_BN));

if q_est(index)*q_BN(index)>0
    q_est = q_est;
else
    q_est = -q_est;
end
